simulink model "NonLinearAirframe"  (R2025a)
settings: Solver=VariableStepAuto  StartTime=0.0  StopTime=10.0  RelTol=1e-3
InitFcn:
  | %% System Constants
  | 
  | %mass
  | m = 1;
  | 
  | %graviational constant
  | g = 9.81;
  | 
  | %Moment of inertia
  | I_XX = 1;
  | I_yy = 1;
  | I_ZZ = 1;
  | 
  | %Torque drag coefficient
  | d_t = 1;
  | 
  | %Distance from CoG to propeller axis
  | l = 1;
  | 
  | %Thrust coefficient
  | b = 1;
  | 
  | %Total rotational moment of inertia around the propeller axis
  | J_TP = 1;
undefined symbols (not defined in the file): I_YY
settings Model: Creator=tobia  LastModifiedBy=tobia

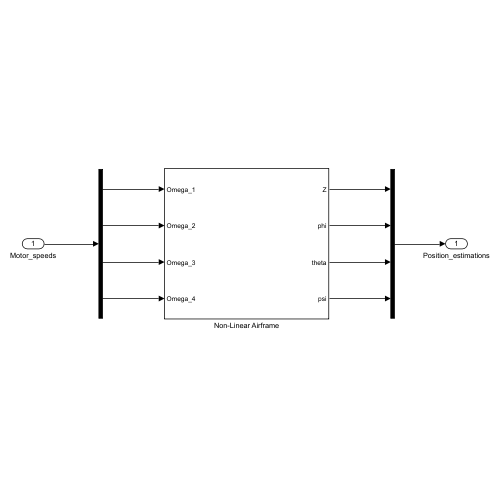
[thumbnail: Simulink's stored preview of the top-level diagram]
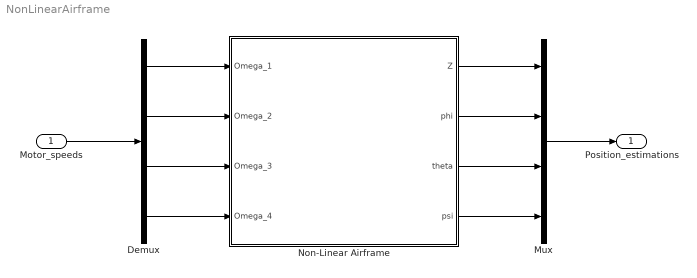
== system NonLinearAirframe ==
  Motor_speeds : Inport
  Demux : Demux
  Mux : Mux
  Non-Linear Airframe : Subsystem
  Position_estimations : Outport
  wires:
  Non-Linear Airframe/4(psi) -> Mux/4
  Non-Linear Airframe/1(Z) -> Mux/1
  Non-Linear Airframe/3(theta) -> Mux/3
  Non-Linear Airframe/2(phi) -> Mux/2
  Mux/1 -> Position_estimations/1
  Demux/2 -> Non-Linear Airframe/2(Omega_2)
  Demux/3 -> Non-Linear Airframe/3(Omega_3)
  Demux/1 -> Non-Linear Airframe/1(Omega_1)
  Motor_speeds/1 -> Demux/1
  Demux/4 -> Non-Linear Airframe/4(Omega_4)

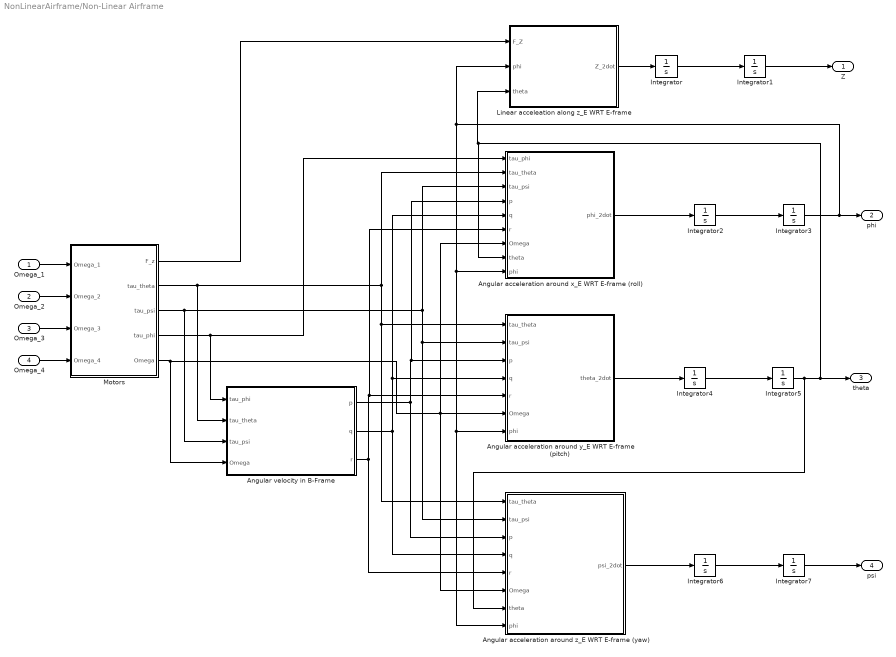
== system NonLinearAirframe/Non-Linear Airframe ==
  Omega_1 : Inport
  Omega_2 : Inport  Port=2
  Omega_3 : Inport  Port=3
  Omega_4 : Inport  Port=4
  Angular acceleration around x_E WRT E-frame (roll) : MATLAB Function  TreatAsAtomicUnit=on
  Angular acceleration around y_E WRT E-frame (pitch) : MATLAB Function  TreatAsAtomicUnit=on
  Angular acceleration around z_E WRT E-frame (yaw) : MATLAB Function  TreatAsAtomicUnit=on
  Angular velocity in B-Frame : Subsystem
  Integrator{,1..7} (8 alike) : Integrator
  Linear acceleation along z_E WRT E-frame : MATLAB Function  TreatAsAtomicUnit=on
  Motors : Subsystem
  Z : Outport
  phi : Outport  Port=2
  theta : Outport  Port=3
  psi : Outport  Port=4
  wires:
  Integrator/1 -> Integrator1/1
  Integrator7/1 -> psi/1
  Motors/1(F_z) -> Linear acceleation along z_E WRT E-frame/1(F_Z)
  Omega_1/1 -> Motors/1(Omega_1)
  Omega_3/1 -> Motors/3(Omega_3)
  Integrator3/1 -> Angular acceleration around z_E WRT E-frame (yaw)/8(phi), Angular acceleration around y_E WRT E-frame (pitch)/7(phi), Angular acceleration around x_E WRT E-frame (roll)/9(phi), Linear acceleation along z_E WRT E-frame/2(phi), phi/1
  Linear acceleation along z_E WRT E-frame/1(Z_2dot) -> Integrator/1
  Omega_4/1 -> Motors/4(Omega_4)
  Integrator6/1 -> Integrator7/1
  Integrator1/1 -> Z/1
  Integrator4/1 -> Integrator5/1
  Integrator2/1 -> Integrator3/1
  Angular acceleration around x_E WRT E-frame (roll)/1(phi_2dot) -> Integrator2/1
  Angular acceleration around y_E WRT E-frame (pitch)/1(theta_2dot) -> Integrator4/1
  Integrator5/1 -> Angular acceleration around z_E WRT E-frame (yaw)/7(theta), theta/1, Angular acceleration around x_E WRT E-frame (roll)/8(theta), Linear acceleation along z_E WRT E-frame/3(theta)
  Omega_2/1 -> Motors/2(Omega_2)
  Angular acceleration around z_E WRT E-frame (yaw)/1(psi_2dot) -> Integrator6/1
  Motors/3(tau_psi) -> Angular velocity in B-Frame/3(tau_psi), Angular acceleration around z_E WRT E-frame (yaw)/2(tau_psi), Angular acceleration around y_E WRT E-frame (pitch)/2(tau_psi), Angular acceleration around x_E WRT E-frame (roll)/3(tau_psi)
  Motors/2(tau_theta) -> Angular velocity in B-Frame/2(tau_theta), Angular acceleration around z_E WRT E-frame (yaw)/1(tau_theta), Angular acceleration around y_E WRT E-frame (pitch)/1(tau_theta), Angular acceleration around x_E WRT E-frame (roll)/2(tau_theta)
  Motors/4(tau_phi) -> Angular acceleration around x_E WRT E-frame (roll)/1(tau_phi), Angular velocity in B-Frame/1(tau_phi)
  Motors/5(Omega) -> Angular acceleration around x_E WRT E-frame (roll)/7(Omega), Angular acceleration around z_E WRT E-frame (yaw)/6(Omega), Angular acceleration around y_E WRT E-frame (pitch)/6(Omega), Angular velocity in B-Frame/4(Omega)
  Angular velocity in B-Frame/3(r) -> Angular acceleration around x_E WRT E-frame (roll)/6(r), Angular acceleration around y_E WRT E-frame (pitch)/5(r), Angular acceleration around z_E WRT E-frame (yaw)/5(r)
  Angular velocity in B-Frame/2(q) -> Angular acceleration around y_E WRT E-frame (pitch)/4(q), Angular acceleration around x_E WRT E-frame (roll)/5(q), Angular acceleration around z_E WRT E-frame (yaw)/4(q)
  Angular velocity in B-Frame/1(p) -> Angular acceleration around x_E WRT E-frame (roll)/4(p), Angular acceleration around y_E WRT E-frame (pitch)/3(p), Angular acceleration around z_E WRT E-frame (yaw)/3(p)

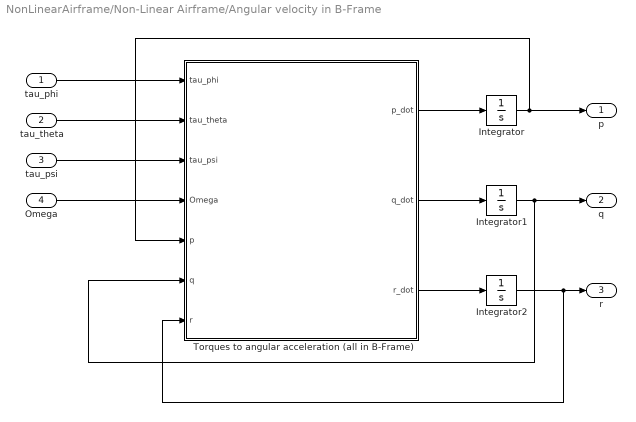
== system NonLinearAirframe/Non-Linear Airframe/Angular velocity in B-Frame ==
  tau_phi : Inport
  tau_theta : Inport  Port=2
  tau_psi : Inport  Port=3
  Omega : Inport  Port=4
  Integrator : Integrator
  Integrator1 : Integrator
  Integrator2 : Integrator
  Torques to angular acceleration (all in B-Frame) : MATLAB Function  TreatAsAtomicUnit=on
  p : Outport
  q : Outport  Port=2
  r : Outport  Port=3
  wires:
  tau_phi/1 -> Torques to angular acceleration (all in B-Frame)/1(tau_phi)
  tau_theta/1 -> Torques to angular acceleration (all in B-Frame)/2(tau_theta)
  tau_psi/1 -> Torques to angular acceleration (all in B-Frame)/3(tau_psi)
  Omega/1 -> Torques to angular acceleration (all in B-Frame)/4(Omega)
  Torques to angular acceleration (all in B-Frame)/3(r_dot) -> Integrator2/1
  Torques to angular acceleration (all in B-Frame)/2(q_dot) -> Integrator1/1
  Torques to angular acceleration (all in B-Frame)/1(p_dot) -> Integrator/1
  Integrator/1 -> Torques to angular acceleration (all in B-Frame)/5(p), p/1
  Integrator1/1 -> Torques to angular acceleration (all in B-Frame)/6(q), q/1
  Integrator2/1 -> Torques to angular acceleration (all in B-Frame)/7(r), r/1

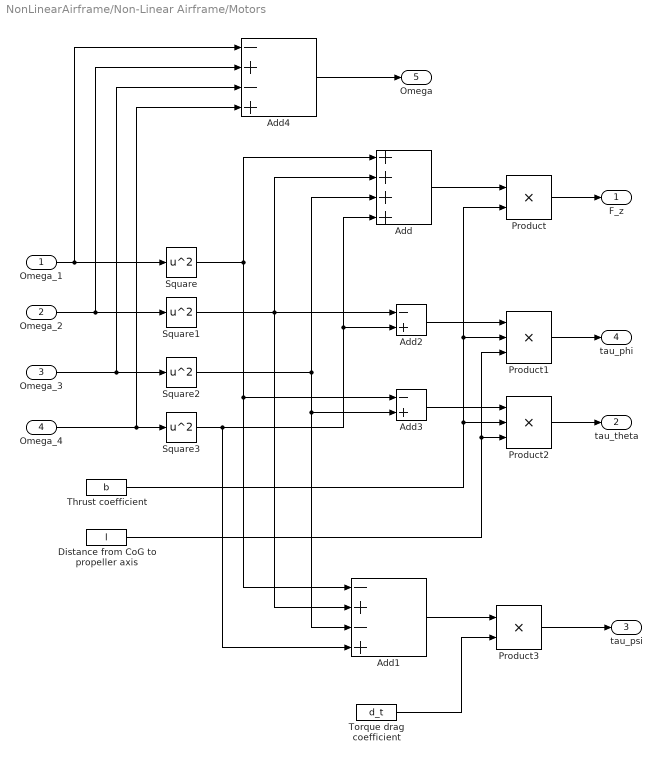
== system NonLinearAirframe/Non-Linear Airframe/Motors ==
  Omega_1 : Inport
  Omega_2 : Inport  Port=2
  Omega_3 : Inport  Port=3
  Omega_4 : Inport  Port=4
  Add : Sum  Inputs=++++
  Add1 : Sum  Inputs=-+-+
  Add2 : Sum  Inputs=-+
  Add3 : Sum  Inputs=-+
  Add4 : Sum  Inputs=-+-+
  Distance from CoG to propeller axis : Constant  Value=l
  Product : Product
  Product1 : Product  Inputs=3
  Product2 : Product  Inputs=3
  Product3 : Product
  Square{,1..3} (4 alike) : Math  Operator=square
  Thrust coefficient : Constant  Value=b
  Torque drag coefficient : Constant  Value=d_t
  F_z : Outport
  tau_theta : Outport  Port=2
  tau_psi : Outport  Port=3
  tau_phi : Outport  Port=4
  Omega : Outport  Port=5
  wires:
  Omega_1/1 -> Add4/1, Square/1
  Omega_2/1 -> Add4/2, Square1/1
  Omega_3/1 -> Add4/3, Square2/1
  Omega_4/1 -> Add4/4, Square3/1
  Square3/1 -> Add1/4, Add/4, Add2/2
  Square2/1 -> Add/3, Add1/3, Add3/2
  Square1/1 -> Add1/2, Add2/1, Add/2
  Square/1 -> Add1/1, Add3/1, Add/1
  Add/1 -> Product/1
  Thrust coefficient/1 -> Product2/2, Product1/2, Product/2
  Distance from CoG to propeller axis/1 -> Product1/3, Product2/3
  Torque drag coefficient/1 -> Product3/2
  Add2/1 -> Product1/1
  Add3/1 -> Product2/1
  Add1/1 -> Product3/1
  Product3/1 -> tau_psi/1
  Product/1 -> F_z/1
  Product1/1 -> tau_phi/1
  Product2/1 -> tau_theta/1
  Add4/1 -> Omega/1

== matlab function NonLinearAirframe/Non-Linear Airframe/Angular acceleration around x_E WRT E-frame (roll) ==
  data: tau_phi input; tau_theta input; tau_psi input; p input; q input; r input; Omega input; theta input; phi input; phi_2dot output; I_XX parameter; I_YY parameter; I_ZZ parameter; J_TP parameter
function phi_2dot = fcn(tau_phi, tau_theta, tau_psi, p, q, r, Omega, theta, phi, I_XX, I_YY, I_ZZ, J_TP)

phi_2dot = tau_phi/I_XX + cos(phi)*tan(theta)*(tau_psi/I_ZZ + (p*q*(- I_YY + I_XX))/I_ZZ) + sin(phi)*tan(theta)*(tau_theta/I_YY + (J_TP*Omega*p)/I_YY - (p*r*(- I_ZZ + I_XX))/I_YY) - (J_TP*Omega*q)/I_XX + (q*r*(- I_ZZ + I_YY))/I_XX;

== matlab function NonLinearAirframe/Non-Linear Airframe/Linear acceleation along z_E WRT E-frame ==
  data: Z_2dot output; F_Z input; m parameter; g parameter; phi input; theta input
function Z_2dot = fcn(F_Z, m, g, phi, theta) 

Z_2dot = -g + (cos(theta) * cos(phi)) * (F_Z / m);

%g = graviational constant
%m = mass

== matlab function NonLinearAirframe/Non-Linear Airframe/Angular acceleration around z_E WRT E-frame (yaw) ==
  data: tau_theta input; tau_psi input; p input; q input; r input; Omega input; theta input; phi input; psi_2dot output; I_XX parameter; I_YY parameter; I_ZZ parameter; J_TP parameter
function psi_2dot = fcn(tau_theta, tau_psi, p, q, r, Omega, theta, phi, I_XX, I_YY, I_ZZ, J_TP)

psi_2dot = cos(phi)*cos(theta)*(tau_psi/I_ZZ + (p*q*(- I_YY + I_XX))/I_ZZ) + cos(theta)*sin(phi)*(tau_theta/I_YY + (J_TP*Omega*p)/I_YY - (p*r*(- I_ZZ + I_XX))/I_YY);

== matlab function NonLinearAirframe/Non-Linear Airframe/Angular velocity in B-Frame/Torques to angular acceleration (all in B-Frame) ==
  data: tau_phi input; p_dot output; q_dot output; r_dot output; tau_theta input; tau_psi input; Omega input; p input; q input; r input; I_XX parameter; I_YY parameter; I_ZZ parameter; J_TP parameter
function [p_dot,q_dot,r_dot] = fcn(tau_phi, tau_theta, tau_psi, Omega, p, q, r, I_XX, I_YY, I_ZZ, J_TP)

p_dot = ((I_YY - I_ZZ)/I_XX) * q * r - (J_TP/I_XX) * q * Omega + tau_phi/I_XX;
q_dot = ((I_ZZ - I_XX)/I_YY) * p * r + (J_TP/I_YY) * p * Omega + tau_theta/I_YY;
r_dot = ((I_XX - I_YY)/I_ZZ) * p * q + tau_psi/I_ZZ;

== matlab function NonLinearAirframe/Non-Linear Airframe/Angular acceleration around y_E WRT E-frame (pitch) ==
  data: tau_theta input; tau_psi input; p input; q input; r input; Omega input; phi input; theta_2dot output; I_XX parameter; I_YY parameter; I_ZZ parameter; J_TP parameter
function theta_2dot = fcn(tau_theta, tau_psi, p, q, r, Omega, phi, I_XX, I_YY, I_ZZ, J_TP)

theta_2dot = cos(phi)*(tau_theta/I_YY + (J_TP*Omega*p)/I_YY - (p*r*(- I_ZZ + I_XX))/I_YY) - sin(phi)*(tau_psi/I_ZZ + (p*q*(- I_YY + I_XX))/I_ZZ);
